simulink model "robot"  (Simulink 7.7)
settings: Solver=ode45  StartTime=0.0  StopTime=10  RelTol=1e-3
libraries: simulink_extras x2
Description:
  | Takes as input [m, l2, g]
settings Model: Creator=Tarik  LastModifiedBy=ttosun
settings DebuggingCC: StrictBusMsg=Warning

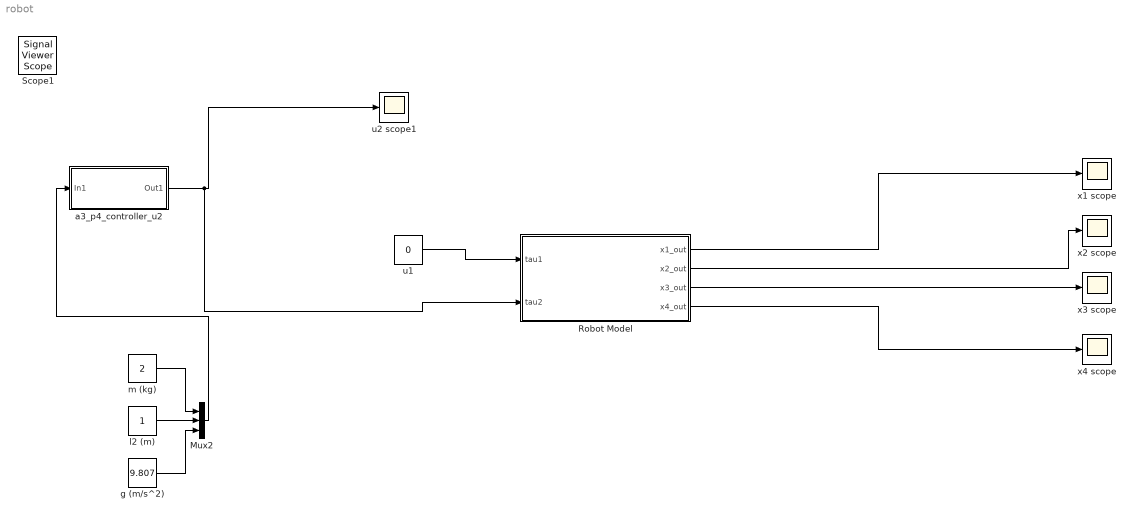
== system robot ==
  Mux2 : Mux  Inputs=3
  Robot Model : Subsystem
  a3_p4_controller_u2 : Subsystem  Description=Input is properties (m l g)
  g (m/s^2) : Constant  Value=9.807
  l2 (m) : Constant
  m (kg) : Constant  Value=2
  u1 : Constant  Value=0
  u2 scope1 : Scope
      settings: TimeRange=20  SaveName=ScopeData4
  x1 scope : Scope
  x2 scope : Scope
  x3 scope : Scope
      settings: TimeRange=20  SaveName=ScopeData2
  x4 scope : Scope
      settings: SaveName=ScopeData3
  Scope1 : SignalViewerScope  IOType=viewer  RefreshTime=0.035000
  wires:
  a3_p4_controller_u2/1(Out1) -> u2 scope1/1, Robot Model/2(tau2)
  Robot Model/1(x1_out) -> x1 scope/1
  Robot Model/2(x2_out) -> x2 scope/1
  Robot Model/3(x3_out) -> x3 scope/1
  Robot Model/4(x4_out) -> x4 scope/1
  u1/1 -> Robot Model/1(tau1)
  m (kg)/1 -> Mux2/1
  l2 (m)/1 -> Mux2/2
  g (m/s^2)/1 -> Mux2/3
  Mux2/1 -> a3_p4_controller_u2/1(In1)

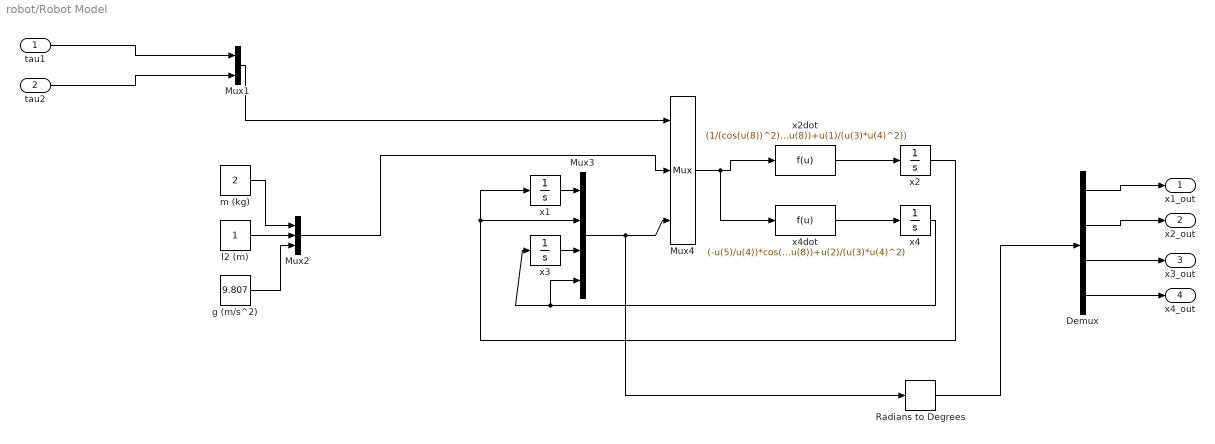
== system robot/Robot Model ==
  tau1 : Inport
  tau2 : Inport  Port=2
  Demux : Demux
  Mux1 : Mux  Inputs=2
  Mux2 : Mux  Inputs=3
  Mux3 : Mux
  Mux4 : Mux  Description=|  Inputs=3
      | u(1:2) are u1 and u2   
      | u(3:5) are m, l2, and g
      | u(6:9) are x1 x2 x3 x4
  Radians to Degrees : simulink_extras/Transformations/Radians to Degrees  SystemSampleTime=-1
  g (m/s^2) : Constant  Value=9.807
  l2 (m) : Constant
  m (kg) : Constant  Value=2
  x1 : Integrator  InitialCondition=-1*pi/180
  x2 : Integrator
  x2dot : Fcn  Expr=(1/(cos(u(8))^2))*(u(7)*u(9)*sin(2*u(8))+u(1)/(u(3)*u(4)^2))
  x3 : Integrator  InitialCondition=-1*pi/180
  x4 : Integrator
  x4dot : Fcn  Expr=(-u(5)/u(4))*cos(u(8))-(u(7)/2)*sin(2*u(8))+u(2)/(u(3)*u(4)^2)
  x1_out : Outport
  x2_out : Outport  Port=2
  x3_out : Outport  Port=3
  x4_out : Outport  Port=4
  wires:
  m (kg)/1 -> Mux2/1
  l2 (m)/1 -> Mux2/2
  g (m/s^2)/1 -> Mux2/3
  x2dot/1 -> x2/1
  x4dot/1 -> x4/1
  Mux3/1 -> Mux4/3, Radians to Degrees/1
  Mux2/1 -> Mux4/2
  Mux1/1 -> Mux4/1
  x3/1 -> Mux3/3
  x4/1 -> Mux3/4, x3/1
  tau1/1 -> Mux1/1
  tau2/1 -> Mux1/2
  Mux4/1 -> x2dot/1, x4dot/1
  x2/1 -> Mux3/2, x1/1
  x1/1 -> Mux3/1
  Demux/1 -> x1_out/1
  Demux/2 -> x2_out/1
  Demux/3 -> x3_out/1
  Demux/4 -> x4_out/1
  Radians to Degrees/1 -> Demux/1

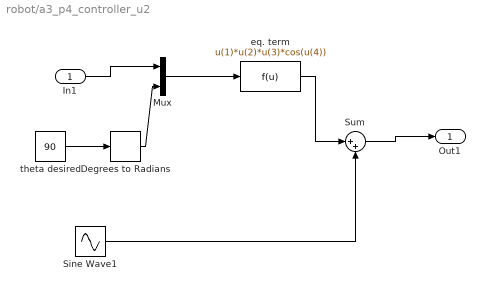
== system robot/a3_p4_controller_u2 ==
  In1 : Inport  PortDimensions=3
  Degrees to Radians : simulink_extras/Transformations/Degrees to Radians  SystemSampleTime=-1
  Mux : Mux  Inputs=2
  Sine Wave1 : Sin  Amplitude=0.1  Frequency=pi  SampleTime=0
  Sum : Sum  Inputs=|++
  eq. term : Fcn  Expr=u(1)*u(2)*u(3)*cos(u(4))
  theta desired : Constant  Value=90
  Out1 : Outport
  wires:
  Mux/1 -> eq. term/1
  In1/1 -> Mux/1
  theta desired/1 -> Degrees to Radians/1
  Degrees to Radians/1 -> Mux/2
  Sine Wave1/1 -> Sum/2
  Sum/1 -> Out1/1
  eq. term/1 -> Sum/1
